simulink model "ABS"  (R2015a)
settings: Solver=ode45  StartTime=0.0  StopTime=20  RelTol=1e-3
undefined symbols (not defined in the file): g, I, m, R, v0
settings Model: Creator=Admin  LastModifiedBy=Admin

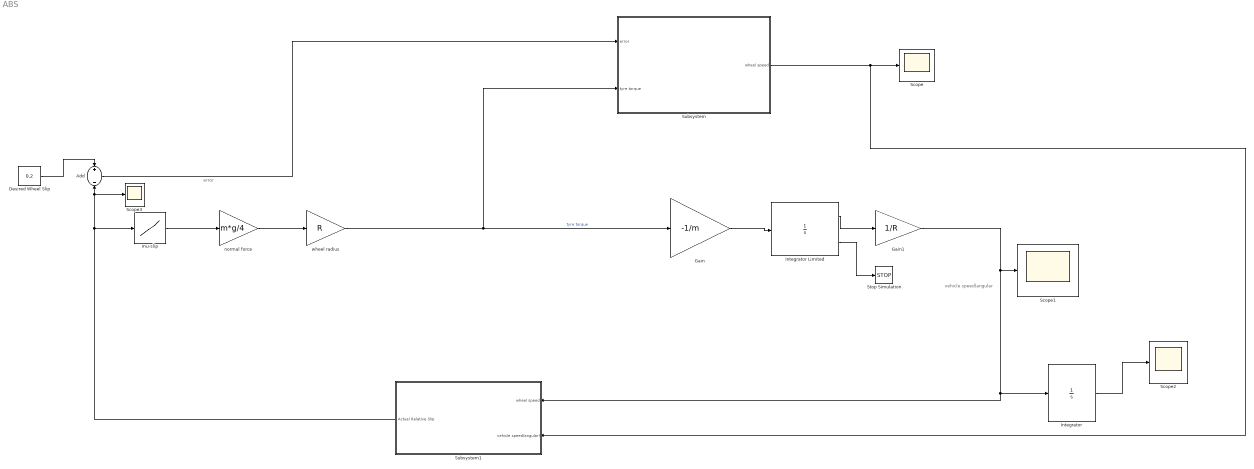
== system ABS ==
  note: error
  note: vehicle speed(angular
  " wheel radius" : Gain  Gain=R
  Add : Sum  Inputs=+-
  Desired Wheel Slip : Constant  Value=0.2
  Gain : Gain  Gain=-1/m
  Gain1 : Gain  Gain=1/R
  Integrator : Integrator
  Integrator Limited : Integrator  InitialCondition=v0  LimitOutput=on  UpperSaturationLimit=1000  LowerSaturationLimit=1  ShowSaturationPort=on
  Scope{,1..3} (4 alike) : Scope
      Scope2 settings: SaveName=ScopeData2
      Scope3 settings: SaveName=ScopeData3
  Stop Simulation : Stop
  Subsystem : Subsystem
  Subsystem1 : Subsystem
  mu-slip : Lookup_n-D  NumberOfTableDimensions=1  BreakpointsForDimension1=[0,0.05,0.1,0.15,0.2,0.25,0.3,0.35,0.4,0.45,0.5,0.55,0.6,0.65,0.7,0.75,0.8,0.85,0.9,0.95,1]  Table=[0,0.4,0.97,0.97,1,0.98,0.96,0.94,0.92,0.9,0.88,0.855,0.83,0.81,0.79,0.77,0.75,0.73,0.72,0.71,0.7]  InternalRulePriority=Speed  RndMeth=Simplest  InputSameDT=on
  normal force : Gain  Gain=m*g/4
  wires:
  Desired Wheel Slip/1 -> Add/1
  normal force/1 -> " wheel radius"/1
  mu-slip/1 -> normal force/1
  Add/1 -> Subsystem/1(error)
  " wheel radius"/1 -> Subsystem/2(tyre torque), Gain/1  "tyre torque"
  Gain/1 -> Integrator Limited/1
  Integrator Limited/1 -> Gain1/1
  Integrator/1 -> Scope2/1
  Gain1/1 -> Subsystem1/1(wheel speed), Integrator/1, Scope1/1
  Subsystem/1(wheel speed) -> Subsystem1/2(vehicle speed(angular)), Scope/1
  Subsystem1/1(Actual Relative Slip) -> mu-slip/1, Scope3/1, Add/2
  Integrator Limited/2 -> Stop Simulation/1

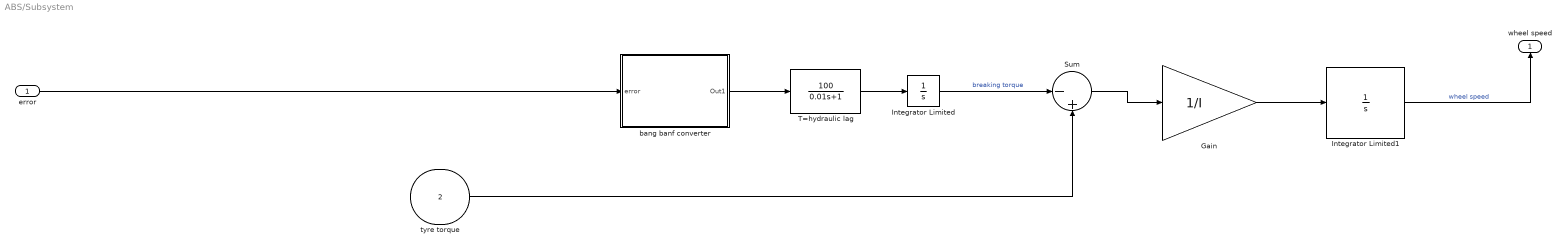
== system ABS/Subsystem ==
  error : Inport
  tyre torque : Inport  Port=2
  Gain : Gain  Gain=1/I
  Integrator Limited : Integrator  LimitOutput=on  UpperSaturationLimit=1000  LowerSaturationLimit=0
  Integrator Limited1 : Integrator  InitialCondition=v0/R  LimitOutput=on  UpperSaturationLimit=1000  LowerSaturationLimit=0
  Sum : Sum  Inputs=|-+
  T=hydraulic lag : TransferFcn  Numerator=[100]  Denominator=[0.01 1]
  bang banf converter : Subsystem
  wheel speed : Outport
  wires:
  Gain/1 -> Integrator Limited1/1
  Integrator Limited1/1 -> wheel speed/1  "wheel speed"
  bang banf converter/1(Out1) -> T=hydraulic lag/1
  error/1 -> bang banf converter/1(error)
  tyre torque/1 -> Sum/2
  T=hydraulic lag/1 -> Integrator Limited/1
  Sum/1 -> Gain/1
  Integrator Limited/1 -> Sum/1  "breaking torque"

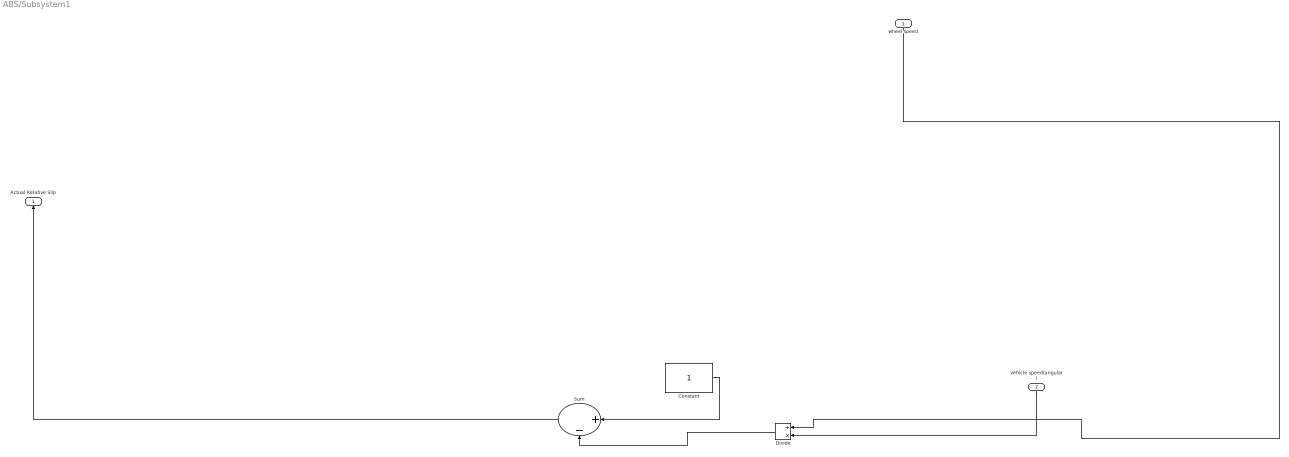
== system ABS/Subsystem1 ==
  wheel speed : Inport
  vehicle speed(angular) : Inport  Port=2
  Constant : Constant
  Divide : Product  Inputs=/*
  Sum : Sum  Inputs=|+-
  Actual Relative Slip : Outport
  wires:
  Sum/1 -> Actual Relative Slip/1
  Constant/1 -> Sum/1
  wheel speed/1 -> Divide/1
  vehicle speed(angular)/1 -> Divide/2
  Divide/1 -> Sum/2

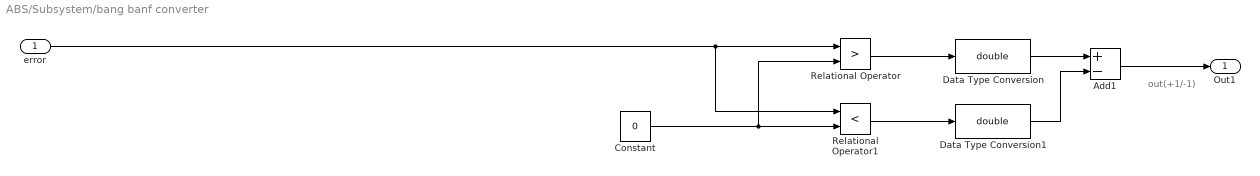
== system ABS/Subsystem/bang banf converter ==
  note: out(+1/-1)
  error : Inport
  Add1 : Sum  Inputs=+-
  Constant : Constant  Value=0
  Data Type Conversion : DataTypeConversion  OutDataTypeStr=double  RndMeth=Zero
  Data Type Conversion1 : DataTypeConversion  OutDataTypeStr=double  RndMeth=Zero
  Relational Operator : RelationalOperator  Operator=>  OutDataTypeStr=boolean
  Relational Operator1 : RelationalOperator  Operator=<  OutDataTypeStr=boolean
  Out1 : Outport
  wires:
  Relational Operator/1 -> Data Type Conversion/1
  Add1/1 -> Out1/1
  Data Type Conversion1/1 -> Add1/2
  error/1 -> Relational Operator1/1, Relational Operator/1
  Constant/1 -> Relational Operator/2, Relational Operator1/2
  Data Type Conversion/1 -> Add1/1
  Relational Operator1/1 -> Data Type Conversion1/1
